simulink model "slexSVMIonospherePredictExample"  (R2021a)
settings: Solver=FixedStepDiscrete  StartTime=0.0  StopTime=radarReturnInput.time(end)  FixedStep=1  RelTol=1e-3
PreLoadFcn:
  | load(fullfile(matlabroot,'help','toolbox','stats','examples','radarReturnInput.mat'))
settings Model: Creator=The MathWorks, Inc.  LastModifiedBy=The MathWorks, Inc.
settings SolverCC: AlgebraicLoopSolver=TrustRegion
settings DataIOCC: ExternalInput=radarReturnInput  LoadExternalInput=on  ReturnWorkspaceOutputs=off  SignalLoggingName=svmlogsout
settings OptimizationCC: DefaultParameterBehavior=Inlined  LifeSpan=inf  EfficientTunableParamExpr=on
settings DebuggingCC: ParameterTunabilityLossMsg=error  SFExecutionAtInitializationDiag=none  SFMachineParentedDataDiag=warning  ArithmeticOperatorsInVariantConditions=warning
settings SFSimCC: SimUseLocalCustomCode=off  CompileTimeRecursionLimit=0  EnableRuntimeRecursion=off  MATLABDynamicMemAlloc=off
settings RTWCC: SystemTargetFile=ert.tlc  TemplateMakefile=ert_default_tmf  GenerateReport=on  RTWUseLocalCustomCode=off  IncludeHyperlinkInReport=on  LaunchReport=on  GenerateTraceInfo=on  GenerateTraceReport=on  GenerateTraceReportSl=on  GenerateTraceReportSf=on  GenerateTraceReportEml=on
settings CodeAppCC: ForceParamTrailComments=on  IgnoreCustomStorageClasses=off  OperatorAnnotations=on  SimulinkDataObjDesc=on  SFDataObjDesc=on  MATLABFcnDesc=on  InsertBlockDesc=on  StateflowObjectComments=on  MATLABSourceComments=on
settings ERTTargetCC: TargetLangStandard=C99 (ISO)  MultiwordLength=2048  GenerateSampleERTMain=on  SupportVariableSizeSignals=on  InlinedParameterPlacement=NonHierarchical  ERTCustomFileTemplate=example_file_process.tlc
settings ConfigComp: CovMetricSettings=dswe

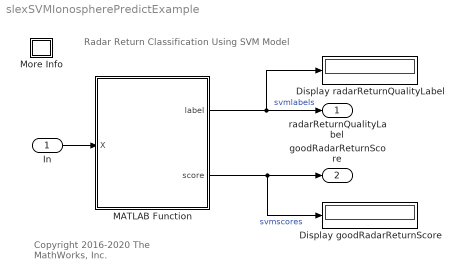
== system slexSVMIonospherePredictExample ==
  note: Radar Return Classification Using SVM Model
  note: Copyright 2016-2020 The MathWorks, Inc.
  In : Inport  PortDimensions=[34]
  Display goodRadarReturnScore : Display
  Display radarReturnQualityLabel : Display
  MATLAB Function : MATLAB Function  TreatAsAtomicUnit=on
  More Info : Subsystem
      settings: OpenFcn=showExample('stats/PredictClassLabelsUsingMATLABFunctionBlockExample')
      mask Display: disp('?')
  radarReturnQualityLabel : Outport  VectorParamsAs1DForOutWhenUnconnected=off
  goodRadarReturnScore : Outport  Port=2  VectorParamsAs1DForOutWhenUnconnected=off
  wires:
  In/1 -> MATLAB Function/1(X)
  MATLAB Function/1(label) -> Display radarReturnQualityLabel/1, radarReturnQualityLabel/1  "svmlabels"
  MATLAB Function/2(score) -> Display goodRadarReturnScore/1, goodRadarReturnScore/1  "svmscores"

== system slexSVMIonospherePredictExample/More Info ==

== matlab function slexSVMIonospherePredictExample/MATLAB Function ==
  data: label output; X input size=[1,34]; score output
function [label,score] = svmIonospherePredict(X) %#codegen
%svmIonospherePredict Predict radar-return quality using SVM model
%   svmIonospherePredict predicts labels and estimates classification
%   scores of the radar returns in the numeric matrix of preditor data X
%   using the compact SVM model in the file SVMIonosphere.mat.  Rows of X
%   correspond to observations and columns to predictor variables.  label
%   is the predicted label and score is the confidence measure for
%   classifying the radar-return quality as good.
%
% Copyright 2016 The MathWorks Inc.
Mdl = loadLearnerForCoder('SVMIonosphere');
[label,bothscores] = predict(Mdl,X);
score = bothscores(:,2);
end
